simulink model "KalmanFilterMWs"  (R2018a)
settings: Solver=VariableStepAuto  StartTime=0.0  StopTime=10.0  RelTol=1e-3
values from neighbouring files (symbols this model uses):
  A = [1 0;     k/m b/m]    [Kalman.m]    (also in fcn.m = [0 1;     -k/m -b/m]; temtProp.m = [0 1;-g/l 0]; untitled2.m = [0 1;     -k/m -b/m])
  B = [0; 1]    [Kalman.m]    (also in fcn.m = [0; 1/m]; temtProp.m = [0;1/(m*l^2)]; untitled2.m = [0; 1/m])
  C = [1 0]    [Kalman.m]    (also in fcn.m = [0 1]; temtProp.m; untitled2.m = [0 1])
  p_pri = A*p_zero*A'    [Kalman.m]    (also in fcn.m = A*p*A + Q)
  R = 1    [Kalman.m]    (also in fcn.m = 0.0001; temtProp.m = 0.0001; untitled2.m = 1-e4)
  x_hzero = [13; 1]    [Kalman.m]    (also in fcn.m = [10; 0]; untitled2.m = [5; 0])
settings Model: Creator=Ali  LastModifiedBy=Ali

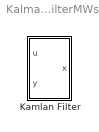
== system KalmanFilterMWs ==
  Kamlan Filter : Subsystem

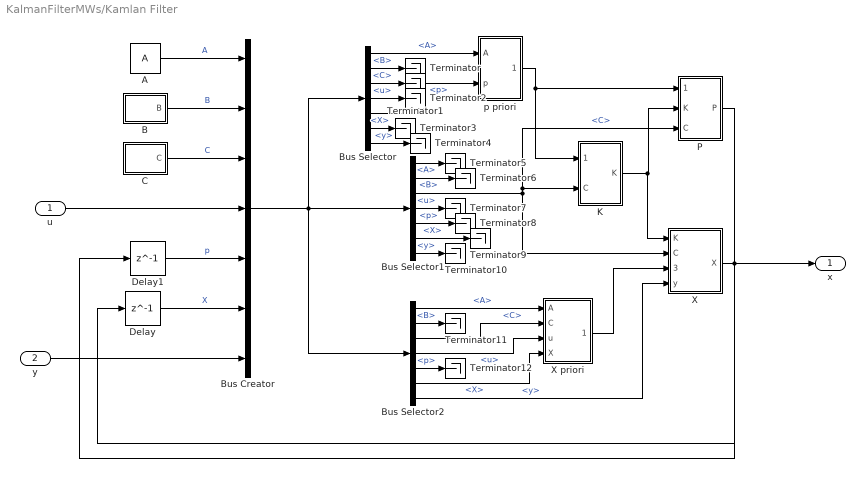
== system KalmanFilterMWs/Kamlan Filter ==
  u : Inport
  y : Inport  Port=2
  A : Constant  Value=A
  B : Subsystem
  Bus Creator : BusCreator  Inputs=7
  Bus Selector : BusSelector  OutputSignals=A,B,C,u,p,X,y
  Bus Selector1 : BusSelector  OutputSignals=A,B,C,u,p,X,y
  Bus Selector2 : BusSelector  OutputSignals=A,B,C,u,p,X,y
  C : Subsystem
  Delay : Delay  DelayLength=1  InitialCondition=x_hzero
  Delay1 : Delay  DelayLength=1  InitialCondition=p_pri
  K : Subsystem
  P : Subsystem
  Terminator{,1..12} (13 alike) : Terminator
  X : Subsystem
  X priori : Subsystem
  p priori : Subsystem
  x : Outport
  wires:
  y/1 -> Bus Creator/7
  Bus Selector/2 -> Terminator/1  "<B>"
  Bus Selector1/6 -> Terminator9/1  "<X>"
  Bus Selector1/2 -> Terminator6/1  "<B>"
  Bus Selector1/5 -> Terminator8/1  "<p>"
  Bus Selector2/7 -> X/4(y)  "<y>"
  B/1(B) -> Bus Creator/2  "B"
  Bus Selector2/1 -> X priori/1(A)  "<A>"
  p priori/1(p priori) -> K/1(p priori), P/1(p priori)
  C/1(C) -> Bus Creator/3  "C"
  Bus Selector/3 -> Terminator1/1  "<C>"
  Bus Selector/5 -> p priori/2(p)  "<p>"
  Bus Selector/4 -> Terminator2/1  "<u>"
  Bus Selector/1 -> p priori/1(A)  "<A>"
  Delay1/1 -> Bus Creator/5  "p"
  Bus Selector2/3 -> X priori/2(C)  "<C>"
  Bus Selector/7 -> Terminator4/1  "<y>"
  Delay/1 -> Bus Creator/6  "X"
  Bus Selector1/7 -> Terminator10/1  "<y>"
  X/1(X) -> x/1, Delay/1
  Bus Creator/1 -> Bus Selector/1, Bus Selector2/1, Bus Selector1/1
  Bus Selector/6 -> Terminator3/1  "<X>"
  Bus Selector1/4 -> Terminator7/1  "<u>"
  Bus Selector2/4 -> X priori/3(u)  "<u>"
  P/1(P) -> Delay1/1
  Bus Selector1/3 -> K/2(C), P/3(C), X/2(C)  "<C>"
  Bus Selector2/2 -> Terminator11/1  "<B>"
  u/1 -> Bus Creator/4
  K/1(K) -> X/1(K), P/2(K)
  Bus Selector1/1 -> Terminator5/1  "<A>"
  A/1 -> Bus Creator/1  "A"
  X priori/1(X priori) -> X/3(X priori)
  Bus Selector2/6 -> X priori/4(X)  "<X>"
  Bus Selector2/5 -> Terminator12/1  "<p>"

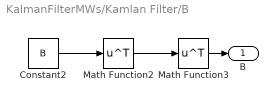
== system KalmanFilterMWs/Kamlan Filter/B ==
  Constant2 : Constant  Value=B
  Math Function2 : Math  Operator=transpose  SaturateOnIntegerOverflow=on
  Math Function3 : Math  Operator=transpose  SaturateOnIntegerOverflow=on
  B : Outport
  wires:
  Math Function3/1 -> B/1
  Math Function2/1 -> Math Function3/1
  Constant2/1 -> Math Function2/1

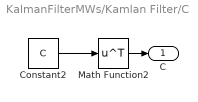
== system KalmanFilterMWs/Kamlan Filter/C ==
  Constant2 : Constant  Value=C
  Math Function2 : Math  Operator=transpose  SaturateOnIntegerOverflow=on
  C : Outport
  wires:
  Math Function2/1 -> C/1
  Constant2/1 -> Math Function2/1

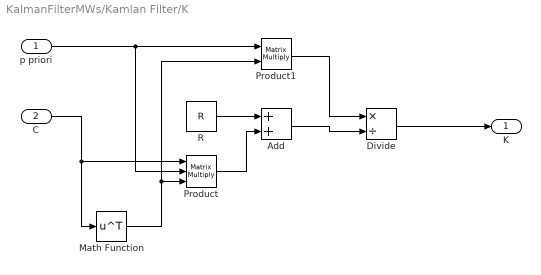
== system KalmanFilterMWs/Kamlan Filter/K ==
  p priori : Inport
  C : Inport  Port=2
  Add : Sum
  Divide : Product  Inputs=*/
  Math Function : Math  Operator=transpose  SaturateOnIntegerOverflow=on
  Product : Product  Inputs=3  Multiplication=Matrix(*)
  Product1 : Product  Multiplication=Matrix(*)
  R : Constant  Value=R
  K : Outport
  wires:
  Product1/1 -> Divide/1
  Product/1 -> Add/2
  Add/1 -> Divide/2
  R/1 -> Add/1
  Divide/1 -> K/1
  p priori/1 -> Product/2, Product1/1
  C/1 -> Math Function/1, Product/1
  Math Function/1 -> Product1/2, Product/3

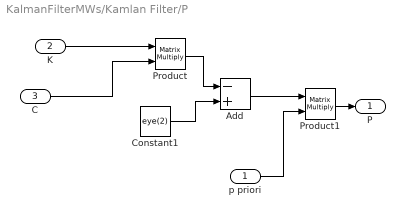
== system KalmanFilterMWs/Kamlan Filter/P ==
  p priori : Inport
  K : Inport  Port=2
  C : Inport  Port=3
  Add : Sum  Inputs=-+
  Constant1 : Constant  Value=eye(2)
  Product : Product  Multiplication=Matrix(*)
  Product1 : Product  Multiplication=Matrix(*)
  P : Outport
  wires:
  C/1 -> Product/2
  Product1/1 -> P/1
  Constant1/1 -> Add/2
  p priori/1 -> Product1/2
  Product/1 -> Add/1
  K/1 -> Product/1
  Add/1 -> Product1/1

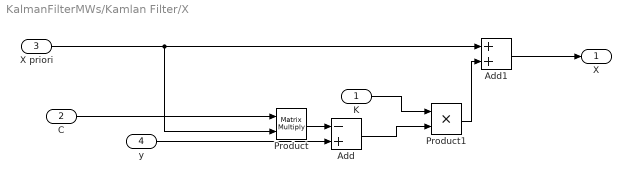
== system KalmanFilterMWs/Kamlan Filter/X ==
  K : Inport
  C : Inport  Port=2
  X priori : Inport  Port=3
  y : Inport  Port=4
  Add : Sum  Inputs=-+
  Add1 : Sum
  Product : Product  Multiplication=Matrix(*)
  Product1 : Product
  X : Outport
  wires:
  K/1 -> Product1/1
  Product1/1 -> Add1/2
  C/1 -> Product/1
  Add1/1 -> X/1
  y/1 -> Add/2
  Add/1 -> Product1/2
  X priori/1 -> Add1/1, Product/2
  Product/1 -> Add/1

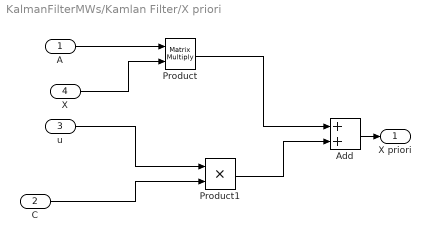
== system KalmanFilterMWs/Kamlan Filter/X priori ==
  A : Inport
  C : Inport  Port=2
  u : Inport  Port=3
  X : Inport  Port=4
  Add : Sum
  Product : Product  Multiplication=Matrix(*)
  Product1 : Product
  X priori : Outport
  wires:
  Add/1 -> X priori/1
  X/1 -> Product/2
  Product1/1 -> Add/2
  C/1 -> Product1/2
  A/1 -> Product/1
  u/1 -> Product1/1
  Product/1 -> Add/1

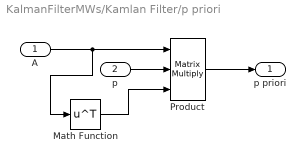
== system KalmanFilterMWs/Kamlan Filter/p priori ==
  A : Inport
  p : Inport  Port=2
  Math Function : Math  Operator=transpose  SaturateOnIntegerOverflow=on
  Product : Product  Inputs=3  Multiplication=Matrix(*)
  p priori : Outport
  wires:
  p/1 -> Product/2
  Product/1 -> p priori/1
  Math Function/1 -> Product/3
  A/1 -> Math Function/1, Product/1
